simulink model "DrivetrainHevIps"  (R2019b)
settings: Solver=VariableStepAuto  StartTime=0.0  StopTime=inf  RelTol=1e-3  EnableMultiTasking=on
model workspace (MAT data in the model file):
  DiffRatio = 3.267
  Jc1 = 0.2
  Jp1 = 0.01
  Jr1 = 0.03
  Js1 = 0.01
  NF = Simulink.Parameter
  NF.Value = 2
  NF.DataType = 'auto'
  NF.Dimensions = [1 1]
  NR = Simulink.Parameter
  NR.Value = 2
  NR.DataType = 'auto'
  NR.Dimensions = [1 1]
  Np1 = 23
  Np2 = 18
  Nr1 = 78
  Nr2 = 58
  Ns1 = 30
  Ns2 = 22
  RWheel = 0.31075
  b_axle = Simulink.Parameter
  b_axle.Value = 10
  b_axle.DataType = 'auto'
  b_axle.Dimensions = [1 1]
  b_driveshaft = Simulink.Parameter
  b_driveshaft.Value = 10
  b_driveshaft.DataType = 'auto'
  b_driveshaft.Dimensions = [1 1]
  bc1 = 0.005
  bp1 = 0.005
  br1 = 0.005
  bs1 = 0.005
  k_axle = Simulink.Parameter
  k_axle.Value = 5000
  k_axle.DataType = 'auto'
  k_axle.Dimensions = [1 1]
  k_driveshaft = Simulink.Parameter
  k_driveshaft.Value = 1000
  k_driveshaft.DataType = 'auto'
  k_driveshaft.Dimensions = [1 1]
  wc_shaft = Simulink.Parameter
  wc_shaft.Value = 50
  wc_shaft.DataType = 'auto'
  wc_shaft.Dimensions = [1 1]
libraries: autolibsharedcoupling x7, autolibpowerinfoutils x6, autolibshareddiff x4, autolibshared x3, autolibcoupling x2
(part 1 of 3)
settings Model: ModifiedByFormat=The MathWorks, Inc.  SimulationMode=accelerator  PauseTimes=10  Creator=The MathWorks, Inc.  LastModifiedBy=The MathWorks, Inc.
settings SolverCC: DecoupledContinuousIntegration=on
settings DataIOCC: DSMLogging=off  ReturnWorkspaceOutputs=off
settings DebuggingCC: ArithmeticOperatorsInVariantConditions=warning
settings ModelReferenceCC: PropagateSignalLabelsOutOfModel=off
settings SFSimCC: SimUseLocalCustomCode=off  CustomCodeUndefinedFunction=UseInterfaceOnly
settings RTWCC: RTWUseLocalCustomCode=off
settings CodeAppCC: StateflowObjectComments=on
settings GRTTargetCC: TargetLangStandard=C89/C90 (ANSI)
settings ConfigComp: CovMetricSettings=dsw  CovHtmlReporting=on  CovSaveCumulativeToWorkspaceVar=on  CovSaveSingleToWorkspaceVar=on  CovShowResultsExplorer=off  CovExternalEMLEnable=off
settings SimscapeCC: SimscapeNormalizeSystem=off  SimscapeNominalValues={1, 'bar'; 1, 'cm^3/s'; 1, 'bar*kg/s'; 1, 'kJ/kg'; 1, 'kW'; }

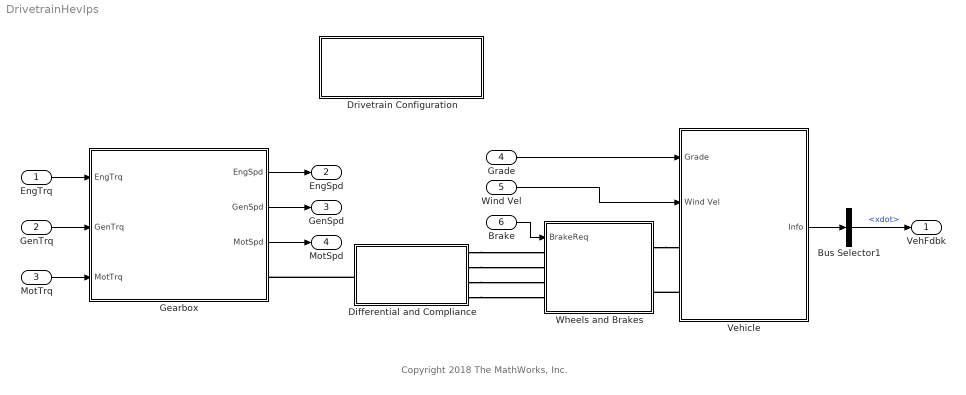
== system DrivetrainHevIps ==
  note: Copyright 2018 The MathWorks, Inc.
  EngTrq : Inport
  GenTrq : Inport  Port=2
  MotTrq : Inport  Port=3
  Grade : Inport  Port=4
  Wind Vel : Inport  Port=5
  Brake : Inport  Port=6
  Bus Selector1 : BusSelector  OutputSignals=BdyFrm.Cg.Vel.xdot
  Differential and Compliance : Subsystem  VariantControlMode=Label  Variant=on  LabelModeActiveChoice=0
  Drivetrain Configuration : Subsystem  mask(Drivetrain Configuration){drivetrainMode=Front Wheel Drive}
      mask prompts: drivetrainMode "Drivetrain Mode"
      mask help: Use this block to configure the dirvetrain mode.
      settings: AttributesFormatString=Active Mode: %<drivetrainMode>
      mask TypeOptions drivetrainMode: Front Wheel Drive | Rear Wheel Drive | All Wheel Drive
      mask Callback drivetrainMode:
      | switch get_param(gcb,'drivetrainMode')
      |     case 'Front Wheel Drive'
      |         set_param([bdroot '/Differential and Compliance'],'OverrideUsingVariant','0')
      |     case 'Rear Wheel Drive'
      |         set_param([bdroot '/Differential and Compliance'],'OverrideUsingVariant','1')
      |     case 'All Wheel Drive'
      |         set_param([bdroot '/Differential and Compliance'],'OverrideUsingVariant','2')
      |     otherwise
      |         set_param([bdroot '/Differential and Compliance'],'OverrideUsingVariant','0')
      | end
      mask Display: disp('Double click to configure drivetrain')
  Gearbox : Subsystem
  Vehicle : Subsystem
  Wheels and Brakes : Subsystem  VariantControl=0
  VehFdbk : Outport  VectorParamsAs1DForOutWhenUnconnected=off
  EngSpd : Outport  Port=2  VectorParamsAs1DForOutWhenUnconnected=off  BusOutputAsStruct=on
  GenSpd : Outport  Port=3  VectorParamsAs1DForOutWhenUnconnected=off  BusOutputAsStruct=on
  MotSpd : Outport  Port=4  VectorParamsAs1DForOutWhenUnconnected=off  BusOutputAsStruct=on
  wires:
  Brake/1 -> Wheels and Brakes/1(BrakeReq)
  EngTrq/1 -> Gearbox/1(EngTrq)
  GenTrq/1 -> Gearbox/2(GenTrq)
  MotTrq/1 -> Gearbox/3(MotTrq)
  Vehicle/1(Info) -> Bus Selector1/1
  Bus Selector1/1 -> VehFdbk/1  "<xdot>"
  Grade/1 -> Vehicle/1(Grade)
  Wind Vel/1 -> Vehicle/2(Wind Vel)
  Gearbox/1(EngSpd) -> EngSpd/1
  Gearbox/2(GenSpd) -> GenSpd/1
  Gearbox/3(MotSpd) -> MotSpd/1
  connections:
  Differential and Compliance/LConn1 -- Gearbox/RConn1
  Differential and Compliance/RConn3 -- Wheels and Brakes/LConn3
  Differential and Compliance/RConn2 -- Wheels and Brakes/LConn2
  Differential and Compliance/RConn4 -- Wheels and Brakes/LConn4
  Vehicle/LConn2 -- Wheels and Brakes/RConn2
  Wheels and Brakes/RConn1 -- Vehicle/LConn1
  Differential and Compliance/RConn1 -- Wheels and Brakes/LConn1

== system DrivetrainHevIps/Differential and Compliance ==
  All Wheel Drive : Subsystem  VariantControl=2
  Front Wheel Drive : Subsystem  VariantControl=0
  Rear Wheel Drive : Subsystem  VariantControl=1
  D : PMIOPort  Side=Left
  FA1 : PMIOPort  Port=2  Side=Right
  FA2 : PMIOPort  Port=3  Side=Right
  RA1 : PMIOPort  Port=4  Side=Right
  RA2 : PMIOPort  Port=5  Side=Right

== system DrivetrainHevIps/Drivetrain Configuration ==

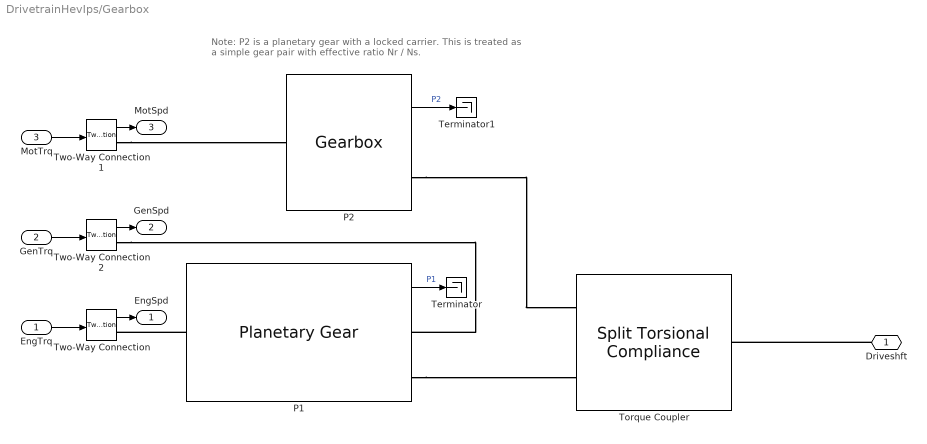
== system DrivetrainHevIps/Gearbox ==
  note: Note: P2 is a planetary gear with a locked carrier.
      | This is treated as a simple gear pair with effective ratio Nr / Ns.
  EngTrq : Inport
  GenTrq : Inport  Port=2
  MotTrq : Inport  Port=3
  P1 : autolibcoupling/Planetary Gear  port_config=Two-way connection  input_config=Torque input - velocity output  Nsp=Ns1/Np1  Nsr=Ns1/Nr1  Js=Js1  Jp=Jp1  Jr=Jr1  Jc=Jc1  bs=bs1  br=br1  bp=bp1  bc=bc1  ws_o=0  wc_o=0  blkID=0
      settings: SourceProductName=Powertrain Blockset  SourceProductBaseCode=PW
  P2 : autolibcoupling/Gearbox  port_config=Two-way connection  input_config=Torque input - velocity output  DiffEffModelPopup=Constant  InterpMethod=Flat  dirSwitch=on  extTamb=off  N=Nr2/Ns2  J1=.01  J2=.01  b1=0.005  b2=0.005  theta1_o=0  w1_o=0  eta=1  eta_tbl=reshape([0.64 0.76 0.8 0.81 0.83 0.84 0.84 0.56 0.73 0.78 0.8 0.83 0.84 0.84 0.54 0.71 0.77 0.8 0.82 0.84 0.84 0.53 0.71 0.77 0.8 0.83 0.84 0.84 0.51 0.71 0.77 0.8 0.83 0.84 0.85 0.52 0.7 0.77 0.8 0.83 0.84 0.85 0.51 0.71 0.76 0.79 0.83 0.84 0.85 0.5 0.69 0.76 0.79 0.82 0.84 0.85 0.45 0.68 0.75 0.78 0.82 0.84 0.85 0.43 0.67 0.74 0.78 0.81 0.83 0.84 0.38 0.63 0.71 0.75 0.8 0.82 0.83 0.81 0.86 0.88 0.89 0.89 0.89 0.9 0.77 0.85 0.87 0.88 0.89 0.9 0.9 0.72 0.82 0.86 0.87 0.88 0.89 0.9 0.68 0.8 0.84 0.86 0.88 0.89 0.89 0.67 0.8 0.84 0.86 0.88 0.89 0.9 0.67 0.8 0.84 0.86 0.88 0.89 0.9 0.65 0.8 0.84 0.86 0.88 0.89 0.9 0.64 0.79 0.83 0.86 0.88 0.89 0.9 0.63 0.78 0.83 0.86 0.88 0.89 0.9 0.59 0.76 0.82 0.85 0.87 0.89 0.9 0.53 0.73 0.8 0.83 0.86 0.88 0.89], 7, 11, 2)  Trq_bpts=[25, 50, 75, 100, 150, 200, 250]  omega_bpts=[52.4 78.5 105 131 157 183 209 262 314 419 524]  Temp_bpts=[290 358]  Tamb=297.15  blkID=0
      settings: SourceProductName=Powertrain Blockset  SourceProductBaseCode=PW
  Terminator : Terminator
  Terminator1 : Terminator
  Torque Coupler : autolibsharedcoupling/Split Torsional Compliance  port_config=Two-way connection  cplrMode=Shaft merge  extInfo=off  k1=k_axle  b1=b_axle  omega1_c=50  theta1_o=0  domega1_o=0  k2=k_axle  b2=b_axle  omega2_c=50  theta2_o=0  domega2_o=0  blkID=0  aMode=1
      settings: SourceProductName=Powertrain Blockset  SourceProductBaseCode=PW
  Two-Way Connection : TwoWayConnection
  Two-Way Connection1 : TwoWayConnection
  Two-Way Connection2 : TwoWayConnection
  Driveshft : PMIOPort  Side=Right
  EngSpd : Outport  VectorParamsAs1DForOutWhenUnconnected=off
  GenSpd : Outport  Port=2  VectorParamsAs1DForOutWhenUnconnected=off
  MotSpd : Outport  Port=3  VectorParamsAs1DForOutWhenUnconnected=off
  wires:
  P2/1 -> Terminator1/1  "P2"
  EngTrq/1 -> Two-Way Connection/1
  Two-Way Connection/1 -> EngSpd/1
  GenTrq/1 -> Two-Way Connection2/1
  P1/1 -> Terminator/1  "P1"
  Two-Way Connection1/1 -> MotSpd/1
  MotTrq/1 -> Two-Way Connection1/1
  Two-Way Connection2/1 -> GenSpd/1
  connections:
  P1/RConn2 -- Torque Coupler/LConn2
  P1/LConn1 -- Two-Way Connection/RConn1
  Two-Way Connection2/RConn1 -- P1/RConn1
  Two-Way Connection1/RConn1 -- P2/LConn1
  P2/RConn1 -- Torque Coupler/LConn1
  Driveshft/RConn1 -- Torque Coupler/RConn1

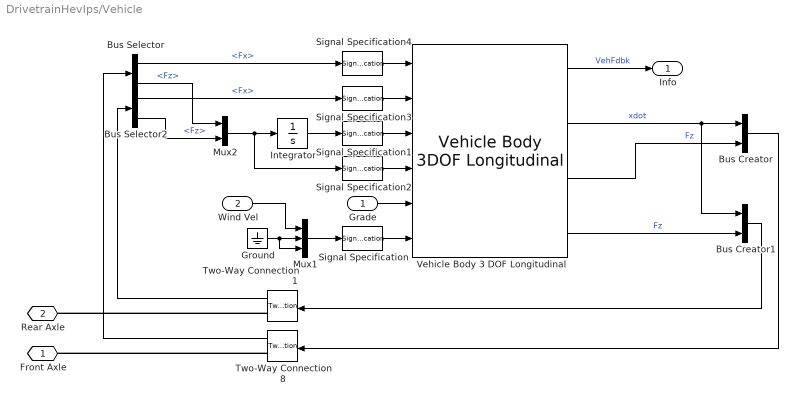
== system DrivetrainHevIps/Vehicle ==
  Grade : Inport  Unit=deg
  Wind Vel : Inport  Port=2  Unit=m/s
  Bus Creator : BusCreator  Inputs=2
  Bus Creator1 : BusCreator  Inputs=2
  Bus Selector : BusSelector  OutputSignals=Fx,Fz
  Bus Selector2 : BusSelector  OutputSignals=Fx,Fz
  Ground : Ground
  Integrator : Integrator
  Mux1 : Mux  Inputs=3
  Mux2 : Mux  Inputs=2
  Signal Specification : SignalSpecification  Unit=m/s
  Signal Specification1 : SignalSpecification  Unit=m
  Signal Specification2 : SignalSpecification  Unit=m/s
  Signal Specification3 : SignalSpecification  Unit=N
  Signal Specification4 : SignalSpecification  Unit=N
  Two-Way Connection1 : TwoWayConnection
  Two-Way Connection8 : TwoWayConnection
  Vehicle Body 3 DOF Longitudinal : autolibshared/Vehicle Body 3DOF Longitudinal  VariantControl=SL  groundType=Axle displacement, velocity  aMode=1  extFMode=off  extMMode=off  extTamb=off  NF=NF  NR=NR  m=1310  a=1.08  b=1.62  h=.5  Cd=0.25  Af=2.27  x_o=0  xdot_o=0  Cl=.1  z_o=-0.298  zdot_o=0  Iyy=3000  Cpm=.1  theta_o=0  q_o=0  FskF=[-50, -1, 0, 2, 3, 52].*1.25e4 / 70  dzsF=[-5e-3, -1e-4, 0, .2, .2001, .2051]  FsbF=[-10000 -100 -10 0 10 100 10000] * 70  dzdotsF=[-10 -1 -.1 0 .1 1 10]  FskR=[-50, -1, 0, 2, 3, 52].*7.5e3 / 70  dzsR=[-5e-3, -1e-4, 0, .2, .2001, .2051]  FsbR=[-10000 -100 -10 0 10 100 10000] * 70  dzdotsR=[-10 -1 -.1 0 .1 1 10]  Pabs=101325  T=273  g=9.81  blkID=0
      settings: SourceProductName=Powertrain Blockset  SourceProductBaseCode=PW
  Front Axle : PMIOPort  Side=Left
  Rear Axle : PMIOPort  Port=2  Side=Left
  Info : Outport  VectorParamsAs1DForOutWhenUnconnected=off
  wires:
  Two-Way Connection1/1 -> Bus Selector2/1
  Bus Selector2/2 -> Mux2/2  "<Fz>"
  Bus Selector2/1 -> Signal Specification3/1  "<Fx>"
  Bus Selector/2 -> Mux2/1  "<Fz>"
  Bus Selector/1 -> Signal Specification4/1  "<Fx>"
  Bus Creator1/1 -> Two-Way Connection1/1
  Bus Creator/1 -> Two-Way Connection8/1
  Signal Specification4/1 -> Vehicle Body 3 DOF Longitudinal/1
  Signal Specification3/1 -> Vehicle Body 3 DOF Longitudinal/2
  Signal Specification2/1 -> Vehicle Body 3 DOF Longitudinal/4
  Signal Specification1/1 -> Vehicle Body 3 DOF Longitudinal/3
  Signal Specification/1 -> Vehicle Body 3 DOF Longitudinal/6
  Grade/1 -> Vehicle Body 3 DOF Longitudinal/5
  Wind Vel/1 -> Mux1/1
  Integrator/1 -> Signal Specification1/1
  Mux2/1 -> Signal Specification2/1, Integrator/1
  Vehicle Body 3 DOF Longitudinal/4 -> Bus Creator1/2  "Fz"
  Mux1/1 -> Signal Specification/1
  Ground/1 -> Mux1/3, Mux1/2
  Vehicle Body 3 DOF Longitudinal/1 -> Info/1  "VehFdbk"
  Two-Way Connection8/1 -> Bus Selector/1
  Vehicle Body 3 DOF Longitudinal/2 -> Bus Creator/1, Bus Creator1/1  "xdot"
  Vehicle Body 3 DOF Longitudinal/3 -> Bus Creator/2  "Fz"
  connections:
  Two-Way Connection1/RConn1 -- Rear Axle/RConn1
  Two-Way Connection8/RConn1 -- Front Axle/RConn1
